simulink model "test_compare"  (R2023a)
settings: Solver=FixedStepAuto  StartTime=0.0  StopTime=10.0  FixedStep=0.002  RelTol=1e-3
PreLoadFcn:
  | xt = importrobot('urdf\XT_PRU_noHands.urdf', 'MaxNumBodies', 25);
  | xt.DataFormat = 'col';
  | 
  | urdfPath = "urdf/XT_PRU_noHands.urdf";
libraries: RoboticsCode x100, robotmaniplib x50
(part 1 of 2)
settings Model: Creator=kgross  LastModifiedBy=speedgoat
settings SolverCC: ConcurrentTasks=on  PositivePriorityOrder=on  AutoInsertRateTranBlk=on
settings OptimizationCC: BlockReduction=off  OptimizeBlockIOStorage=off
settings DebuggingCC: TasksWithSamePriorityMsg=none
settings HardwareCC: ProdBitPerLong=64  ProdLongLongMode=on  ProdHWDeviceType=Intel->x86-64 (Linux 64)
settings SFSimCC: SimTargetLang=C++
settings RTWCC: Description=Simulink Real-Time  SystemTargetFile=slrealtime.tlc  TemplateMakefile=slrealtime_default_tmf  Toolchain=Simulink Real-Time Toolchain  BuildConfiguration=Faster Runs  CodeExecutionProfiling=on  TargetLang=C++

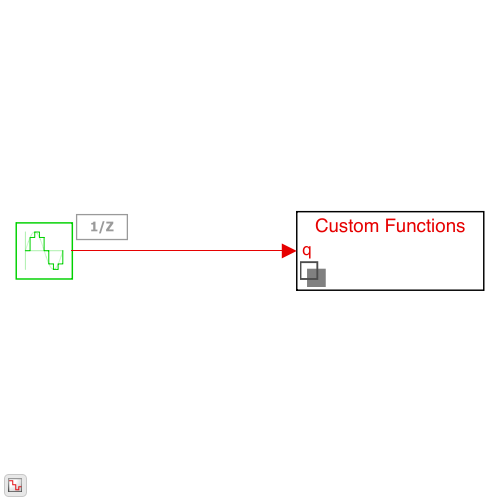
[thumbnail: Simulink's stored preview of the top-level diagram]
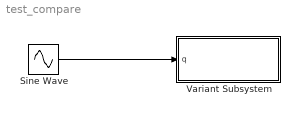
== system test_compare ==
  Sine Wave : Sin  Amplitude=1:16  Frequency=1:16  SampleTime=1
  Variant Subsystem : Subsystem  Variant=on  VariantControlMode=label  LabelModeActiveChoice=Custom
  wires:
  Sine Wave/1 -> Variant Subsystem/1(q)

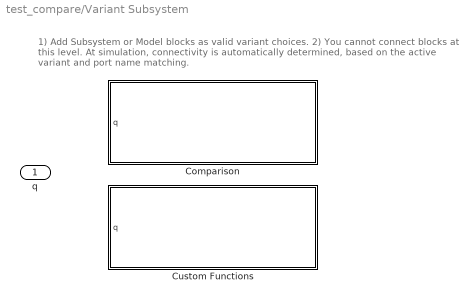
== system test_compare/Variant Subsystem ==
  note: 1) Add Subsystem or Model blocks as valid variant choices.
      | 2) You cannot connect blocks at this level. At simulation, connectivity is automatically
      | determined, based on the active variant and port name matching.
  q : Inport
  Comparison : Subsystem  VariantControl=Comparison
  Custom Functions : Subsystem  VariantControl=Custom

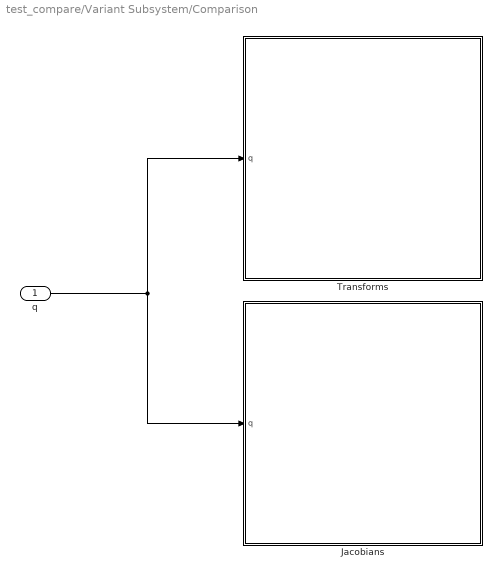
== system test_compare/Variant Subsystem/Comparison ==
  q : Inport
  Jacobians : Subsystem  VariantControl=Choice
  Transforms : Subsystem  VariantControl=Choice_1
  wires:
  q/1 -> Transforms/1(q), Jacobians/1(q)

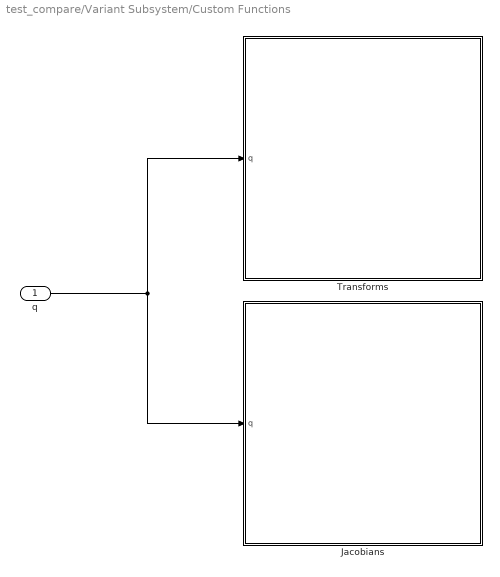
== system test_compare/Variant Subsystem/Custom Functions ==
  q : Inport
  Jacobians : Subsystem  VariantControl=Choice
  Transforms : Subsystem  VariantControl=Choice_1
  wires:
  q/1 -> Jacobians/1(q), Transforms/1(q)

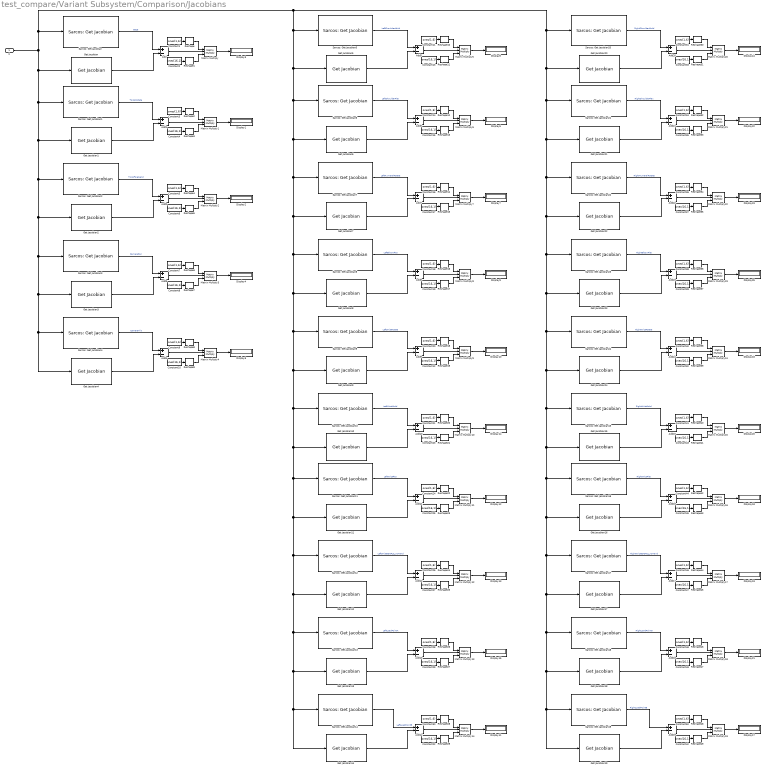
== system test_compare/Variant Subsystem/Comparison/Jacobians ==
  q : Inport
  Add{,1..24} (25 alike) : Sum  Inputs=+-
  Constant{1,3,5,7,9,11,14,16,18,20..21,24,26,28,30..31,34,36,38,40..41,44,46,48,50} (25 alike) : Constant  Value=ones(1,6)
  Constant{2,4,6,8,10,12..13,15,17,19,22..23,25,27,29,32..33,35,37,39,42..43,45,47,49} (25 alike) : Constant  Value=ones(16,1)
  Display{1..25} (25 alike) : Display
  Get Jacobian : robotmaniplib/Get Jacobian  RigidBodyTree=xt  EndEffector=Base  SimulateUsing=Interpreted execution
  Get Jacobian1 : robotmaniplib/Get Jacobian  RigidBodyTree=xt  EndEffector=TorsoRotate  SimulateUsing=Interpreted execution
  Get Jacobian10 : robotmaniplib/Get Jacobian  RigidBodyTree=xt  EndEffector=LeftWristAbAd  SimulateUsing=Interpreted execution
  Get Jacobian11 : robotmaniplib/Get Jacobian  RigidBodyTree=xt  EndEffector=LeftWristFlex  SimulateUsing=Interpreted execution
  Get Jacobian12 : robotmaniplib/Get Jacobian  RigidBodyTree=xt  EndEffector=LeftWrist6DOFLC_noHand  SimulateUsing=Interpreted execution
  Get Jacobian13 : robotmaniplib/Get Jacobian  RigidBodyTree=xt  EndEffector=LeftLoadPointA  SimulateUsing=Interpreted execution
  Get Jacobian14 : robotmaniplib/Get Jacobian  RigidBodyTree=xt  EndEffector=LeftLoadPointB  SimulateUsing=Interpreted execution
  Get Jacobian15 : robotmaniplib/Get Jacobian  RigidBodyTree=xt  EndEffector=RightWristAbAd  SimulateUsing=Interpreted execution
  Get Jacobian16 : robotmaniplib/Get Jacobian  RigidBodyTree=xt  EndEffector=RightWristFlex  SimulateUsing=Interpreted execution
  Get Jacobian17 : robotmaniplib/Get Jacobian  RigidBodyTree=xt  EndEffector=RightWrist6DOFLC_noHand  SimulateUsing=Interpreted execution
  Get Jacobian18 : robotmaniplib/Get Jacobian  RigidBodyTree=xt  EndEffector=RightLoadPointA  SimulateUsing=Interpreted execution
  Get Jacobian19 : robotmaniplib/Get Jacobian  RigidBodyTree=xt  EndEffector=RightLoadPointB  SimulateUsing=Interpreted execution
  Get Jacobian2 : robotmaniplib/Get Jacobian  RigidBodyTree=xt  EndEffector=TorsoForebend  SimulateUsing=Interpreted execution
  Get Jacobian20 : robotmaniplib/Get Jacobian  RigidBodyTree=xt  EndEffector=RightShoulderAbAd  SimulateUsing=Interpreted execution
  Get Jacobian21 : robotmaniplib/Get Jacobian  RigidBodyTree=xt  EndEffector=RightShoulderFlex  SimulateUsing=Interpreted execution
  Get Jacobian22 : robotmaniplib/Get Jacobian  RigidBodyTree=xt  EndEffector=RightHumeralRotate  SimulateUsing=Interpreted execution
  Get Jacobian23 : robotmaniplib/Get Jacobian  RigidBodyTree=xt  EndEffector=RightElbowFlex  SimulateUsing=Interpreted execution
  Get Jacobian24 : robotmaniplib/Get Jacobian  RigidBodyTree=xt  EndEffector=RightWristRotate  SimulateUsing=Interpreted execution
  Get Jacobian3 : robotmaniplib/Get Jacobian  RigidBodyTree=xt  EndEffector=CameraPan  SimulateUsing=Interpreted execution
  Get Jacobian4 : robotmaniplib/Get Jacobian  RigidBodyTree=xt  EndEffector=CameraTilt  SimulateUsing=Interpreted execution
  Get Jacobian5 : robotmaniplib/Get Jacobian  RigidBodyTree=xt  EndEffector=LeftShoulderAbAd  SimulateUsing=Interpreted execution
  Get Jacobian6 : robotmaniplib/Get Jacobian  RigidBodyTree=xt  EndEffector=LeftShoulderFlex  SimulateUsing=Interpreted execution
  Get Jacobian7 : robotmaniplib/Get Jacobian  RigidBodyTree=xt  EndEffector=LeftHumeralRotate  SimulateUsing=Interpreted execution
  Get Jacobian8 : robotmaniplib/Get Jacobian  RigidBodyTree=xt  EndEffector=LeftElbowFlex  SimulateUsing=Interpreted execution
  Get Jacobian9 : robotmaniplib/Get Jacobian  RigidBodyTree=xt  EndEffector=LeftWristRotate  SimulateUsing=Interpreted execution
  Matrix Multiply{,1..24} (25 alike) : Product  Inputs=3  Multiplication=Matrix(*)
  Reshape{,2,4,6,8,10,12,14,16,18,20,22,24,26,28,30,32,34,36,38,40,42,44,46,48} (25 alike) : Reshape  OutputDimensionality=Row vector (2-D)
  Reshape{1,3,5,7,9,11,13,15,17,19,21,23,25,27,29,31,33,35,37,39,41,43,45,47,49} (25 alike) : Reshape  OutputDimensionality=Column vector (2-D)
  Sarcos: Get Jacobian : RoboticsCode/Sarcos: Get Jacobian  urdfpath='XT_PRU_noHands.urdf'  source=Base  source_string='Base'  names_length=16
      settings: SourceProductName=Sacros Robotics Toolbox
  Sarcos: Get Jacobian1 : RoboticsCode/Sarcos: Get Jacobian  urdfpath='XT_PRU_noHands.urdf'  source=TorsoRotate  source_string='TorsoRotate'  names_length=16
      settings: SourceProductName=Sacros Robotics Toolbox
  Sarcos: Get Jacobian10 : RoboticsCode/Sarcos: Get Jacobian  urdfpath='XT_PRU_noHands.urdf'  source=LeftWristAbAd  source_string='LeftWristAbAd'  names_length=16
      settings: SourceProductName=Sacros Robotics Toolbox
  Sarcos: Get Jacobian11 : RoboticsCode/Sarcos: Get Jacobian  urdfpath='XT_PRU_noHands.urdf'  source=LeftWristFlex  source_string='LeftWristFlex'  names_length=16
      settings: SourceProductName=Sacros Robotics Toolbox
  Sarcos: Get Jacobian12 : RoboticsCode/Sarcos: Get Jacobian  urdfpath='XT_PRU_noHands.urdf'  source=LeftWrist6DOFLC_noHand  source_string='LeftWrist6DOFLC_noHand'  names_length=16
      settings: SourceProductName=Sacros Robotics Toolbox
  Sarcos: Get Jacobian13 : RoboticsCode/Sarcos: Get Jacobian  urdfpath='XT_PRU_noHands.urdf'  source=LeftLoadPointA  source_string='LeftLoadPointA'  names_length=16
      settings: SourceProductName=Sacros Robotics Toolbox
  Sarcos: Get Jacobian14 : RoboticsCode/Sarcos: Get Jacobian  urdfpath='XT_PRU_noHands.urdf'  source=LeftLoadPointB  source_string='LeftLoadPointB'  names_length=16
      settings: SourceProductName=Sacros Robotics Toolbox
  Sarcos: Get Jacobian15 : RoboticsCode/Sarcos: Get Jacobian  urdfpath='XT_PRU_noHands.urdf'  source=RightWristAbAd  source_string='RightWristAbAd'  names_length=16
      settings: SourceProductName=Sacros Robotics Toolbox
  Sarcos: Get Jacobian16 : RoboticsCode/Sarcos: Get Jacobian  urdfpath='XT_PRU_noHands.urdf'  source=RightWristFlex  source_string='RightWristFlex'  names_length=16
      settings: SourceProductName=Sacros Robotics Toolbox
  Sarcos: Get Jacobian17 : RoboticsCode/Sarcos: Get Jacobian  urdfpath='XT_PRU_noHands.urdf'  source=RightWrist6DOFLC_noHand  source_string='RightWrist6DOFLC_noHand'  names_length=16
      settings: SourceProductName=Sacros Robotics Toolbox
  Sarcos: Get Jacobian18 : RoboticsCode/Sarcos: Get Jacobian  urdfpath='XT_PRU_noHands.urdf'  source=RightLoadPointA  source_string='RightLoadPointA'  names_length=16
      settings: SourceProductName=Sacros Robotics Toolbox
  Sarcos: Get Jacobian19 : RoboticsCode/Sarcos: Get Jacobian  urdfpath='XT_PRU_noHands.urdf'  source=RightLoadPointB  source_string='RightLoadPointB'  names_length=16
      settings: SourceProductName=Sacros Robotics Toolbox
  Sarcos: Get Jacobian2 : RoboticsCode/Sarcos: Get Jacobian  urdfpath='XT_PRU_noHands.urdf'  source=TorsoForebend  source_string='TorsoForebend'  names_length=16
      settings: SourceProductName=Sacros Robotics Toolbox
  Sarcos: Get Jacobian20 : RoboticsCode/Sarcos: Get Jacobian  urdfpath='XT_PRU_noHands.urdf'  source=RightShoulderAbAd  source_string='RightShoulderAbAd'  names_length=16
      settings: SourceProductName=Sacros Robotics Toolbox
  Sarcos: Get Jacobian21 : RoboticsCode/Sarcos: Get Jacobian  urdfpath='XT_PRU_noHands.urdf'  source=RightShoulderFlex  source_string='RightShoulderFlex'  names_length=16
      settings: SourceProductName=Sacros Robotics Toolbox
  Sarcos: Get Jacobian22 : RoboticsCode/Sarcos: Get Jacobian  urdfpath='XT_PRU_noHands.urdf'  source=RightHumeralRotate  source_string='RightHumeralRotate'  names_length=16
      settings: SourceProductName=Sacros Robotics Toolbox
  Sarcos: Get Jacobian23 : RoboticsCode/Sarcos: Get Jacobian  urdfpath='XT_PRU_noHands.urdf'  source=RightElbowFlex  source_string='RightElbowFlex'  names_length=16
      settings: SourceProductName=Sacros Robotics Toolbox
  Sarcos: Get Jacobian24 : RoboticsCode/Sarcos: Get Jacobian  urdfpath='XT_PRU_noHands.urdf'  source=RightWristRotate  source_string='RightWristRotate'  names_length=16
      settings: SourceProductName=Sacros Robotics Toolbox
  Sarcos: Get Jacobian3 : RoboticsCode/Sarcos: Get Jacobian  urdfpath='XT_PRU_noHands.urdf'  source=CameraPan  source_string='CameraPan'  names_length=16
      settings: SourceProductName=Sacros Robotics Toolbox
  Sarcos: Get Jacobian4 : RoboticsCode/Sarcos: Get Jacobian  urdfpath='XT_PRU_noHands.urdf'  source=CameraTilt  source_string='CameraTilt'  names_length=16
      settings: SourceProductName=Sacros Robotics Toolbox
  Sarcos: Get Jacobian5 : RoboticsCode/Sarcos: Get Jacobian  urdfpath='XT_PRU_noHands.urdf'  source=LeftShoulderAbAd  source_string='LeftShoulderAbAd'  names_length=16
      settings: SourceProductName=Sacros Robotics Toolbox
  Sarcos: Get Jacobian6 : RoboticsCode/Sarcos: Get Jacobian  urdfpath='XT_PRU_noHands.urdf'  source=LeftShoulderFlex  source_string='LeftShoulderFlex'  names_length=16
      settings: SourceProductName=Sacros Robotics Toolbox
  Sarcos: Get Jacobian7 : RoboticsCode/Sarcos: Get Jacobian  urdfpath='XT_PRU_noHands.urdf'  source=LeftHumeralRotate  source_string='LeftHumeralRotate'  names_length=16
      settings: SourceProductName=Sacros Robotics Toolbox
  Sarcos: Get Jacobian8 : RoboticsCode/Sarcos: Get Jacobian  urdfpath='XT_PRU_noHands.urdf'  source=LeftElbowFlex  source_string='LeftElbowFlex'  names_length=16
      settings: SourceProductName=Sacros Robotics Toolbox
  Sarcos: Get Jacobian9 : RoboticsCode/Sarcos: Get Jacobian  urdfpath='XT_PRU_noHands.urdf'  source=LeftWristRotate  source_string='LeftWristRotate'  names_length=16
      settings: SourceProductName=Sacros Robotics Toolbox
  wires:
  Reshape1/1 -> Matrix Multiply/3
  Reshape/1 -> Matrix Multiply/1
  Constant2/1 -> Reshape1/1
  Matrix Multiply/1 -> Display3/1
  Constant1/1 -> Reshape/1
  Get Jacobian/1 -> Add/2
  Sarcos: Get Jacobian/1 -> Add/1  "Base"
  Add/1 -> Matrix Multiply/2
  Add1/1 -> Matrix Multiply1/2
  Sarcos: Get Jacobian1/1 -> Add1/1  "TorsoRotate"
  Get Jacobian1/1 -> Add1/2
  Constant3/1 -> Reshape2/1
  Matrix Multiply1/1 -> Display1/1
  Constant4/1 -> Reshape3/1
  Reshape2/1 -> Matrix Multiply1/1
  Reshape3/1 -> Matrix Multiply1/3
  Reshape5/1 -> Matrix Multiply2/3
  Reshape4/1 -> Matrix Multiply2/1
  Constant6/1 -> Reshape5/1
  Matrix Multiply2/1 -> Display2/1
  Constant5/1 -> Reshape4/1
  Get Jacobian2/1 -> Add2/2
  Sarcos: Get Jacobian2/1 -> Add2/1  "TorsoForebend"
  Add2/1 -> Matrix Multiply2/2
  Add3/1 -> Matrix Multiply3/2
  Sarcos: Get Jacobian3/1 -> Add3/1  "CameraPan"
  Get Jacobian3/1 -> Add3/2
  Constant7/1 -> Reshape6/1
  Matrix Multiply3/1 -> Display4/1
  Constant8/1 -> Reshape7/1
  Reshape6/1 -> Matrix Multiply3/1
  Reshape7/1 -> Matrix Multiply3/3
  Reshape9/1 -> Matrix Multiply4/3
  Reshape8/1 -> Matrix Multiply4/1
  Constant10/1 -> Reshape9/1
  Matrix Multiply4/1 -> Display5/1
  Constant9/1 -> Reshape8/1
  Get Jacobian4/1 -> Add4/2
  Sarcos: Get Jacobian4/1 -> Add4/1  "CameraTilt"
  Add4/1 -> Matrix Multiply4/2
  Add9/1 -> Matrix Multiply9/2
  Sarcos: Get Jacobian9/1 -> Add9/1  "LeftWristRotate"
  Get Jacobian9/1 -> Add9/2
  Constant20/1 -> Reshape18/1
  Matrix Multiply9/1 -> Display10/1
  Constant12/1 -> Reshape19/1
  Reshape18/1 -> Matrix Multiply9/1
  Reshape19/1 -> Matrix Multiply9/3
  Reshape17/1 -> Matrix Multiply8/3
  Reshape16/1 -> Matrix Multiply8/1
  Constant19/1 -> Reshape17/1
  Matrix Multiply8/1 -> Display9/1
  Constant18/1 -> Reshape16/1
  Get Jacobian8/1 -> Add8/2
  Sarcos: Get Jacobian8/1 -> Add8/1  "LeftElbowFlex"
  Add8/1 -> Matrix Multiply8/2
  Add7/1 -> Matrix Multiply7/2
  Sarcos: Get Jacobian7/1 -> Add7/1  "LeftHumeralRotate"
  Get Jacobian7/1 -> Add7/2
  Constant16/1 -> Reshape14/1
  Matrix Multiply7/1 -> Display7/1
  Constant17/1 -> Reshape15/1
  Reshape14/1 -> Matrix Multiply7/1
  Reshape15/1 -> Matrix Multiply7/3
  Reshape13/1 -> Matrix Multiply6/3
  Reshape12/1 -> Matrix Multiply6/1
  Constant15/1 -> Reshape13/1
  Matrix Multiply6/1 -> Display6/1
  Constant14/1 -> Reshape12/1
  Get Jacobian6/1 -> Add6/2
  Sarcos: Get Jacobian6/1 -> Add6/1  "LeftShoulderFlex"
  Add6/1 -> Matrix Multiply6/2
  Add5/1 -> Matrix Multiply5/2
  Sarcos: Get Jacobian5/1 -> Add5/1  "LeftShoulderAbAd"
  Get Jacobian5/1 -> Add5/2
  Constant11/1 -> Reshape10/1
  Matrix Multiply5/1 -> Display8/1
  Constant13/1 -> Reshape11/1
  Reshape10/1 -> Matrix Multiply5/1
  Reshape11/1 -> Matrix Multiply5/3
  Constant30/1 -> Reshape28/1
  Reshape27/1 -> Matrix Multiply13/3
  Get Jacobian14/1 -> Add14/2
  Reshape21/1 -> Matrix Multiply10/3
  Constant21/1 -> Reshape20/1
  Get Jacobian10/1 -> Add10/2
  Constant23/1 -> Reshape21/1
  Sarcos: Get Jacobian10/1 -> Add10/1  "LeftWristAbAd"
  Matrix Multiply10/1 -> Display14/1
  Add11/1 -> Matrix Multiply11/2
  Reshape29/1 -> Matrix Multiply14/3
  Constant24/1 -> Reshape22/1
  Reshape20/1 -> Matrix Multiply10/1
  Sarcos: Get Jacobian11/1 -> Add11/1  "LeftWristFlex"
  Get Jacobian11/1 -> Add11/2
  Constant25/1 -> Reshape23/1
  Reshape24/1 -> Matrix Multiply12/1
  Reshape22/1 -> Matrix Multiply11/1
  Reshape25/1 -> Matrix Multiply12/3
  Reshape23/1 -> Matrix Multiply11/3
  Constant27/1 -> Reshape25/1
  Reshape28/1 -> Matrix Multiply14/1
  Matrix Multiply12/1 -> Display13/1
  Reshape26/1 -> Matrix Multiply13/1
  Add12/1 -> Matrix Multiply12/2
  Get Jacobian12/1 -> Add12/2
  Matrix Multiply11/1 -> Display12/1
  Sarcos: Get Jacobian14/1 -> Add14/1  "LeftLoadPointB"
  Constant22/1 -> Reshape29/1
  Sarcos: Get Jacobian12/1 -> Add12/1  "LeftWrist6DOFLC_noHand"
  Matrix Multiply13/1 -> Display15/1
  Constant28/1 -> Reshape26/1
  Sarcos: Get Jacobian13/1 -> Add13/1  "LeftLoadPointA"
  Matrix Multiply14/1 -> Display11/1
  Get Jacobian13/1 -> Add13/2
  Add14/1 -> Matrix Multiply14/2
  Constant29/1 -> Reshape27/1
  Constant26/1 -> Reshape24/1
  Add13/1 -> Matrix Multiply13/2
  Add10/1 -> Matrix Multiply10/2
  Add15/1 -> Matrix Multiply15/2
  Add18/1 -> Matrix Multiply18/2
  Constant46/1 -> Reshape44/1
  Constant49/1 -> Reshape47/1
  Add19/1 -> Matrix Multiply19/2
  Get Jacobian18/1 -> Add18/2
  Matrix Multiply19/1 -> Display17/1
  Sarcos: Get Jacobian18/1 -> Add18/1  "RightLoadPointA"
  Constant48/1 -> Reshape46/1
  Matrix Multiply18/1 -> Display21/1
  Sarcos: Get Jacobian17/1 -> Add17/1  "RightWrist6DOFLC_noHand"
  Constant42/1 -> Reshape49/1
  Sarcos: Get Jacobian19/1 -> Add19/1  "RightLoadPointB"
  Matrix Multiply16/1 -> Display18/1
  Get Jacobian17/1 -> Add17/2
  Add17/1 -> Matrix Multiply17/2
  Reshape46/1 -> Matrix Multiply18/1
  Matrix Multiply17/1 -> Display19/1
  Reshape48/1 -> Matrix Multiply19/1
  Constant47/1 -> Reshape45/1
  Reshape43/1 -> Matrix Multiply16/3
  Reshape45/1 -> Matrix Multiply17/3
  Reshape42/1 -> Matrix Multiply16/1
  Reshape44/1 -> Matrix Multiply17/1
  Constant45/1 -> Reshape43/1
  Get Jacobian16/1 -> Add16/2
  Sarcos: Get Jacobian16/1 -> Add16/1  "RightWristFlex"
  Reshape40/1 -> Matrix Multiply15/1
  Constant44/1 -> Reshape42/1
  Reshape49/1 -> Matrix Multiply19/3
  Add16/1 -> Matrix Multiply16/2
  Matrix Multiply15/1 -> Display20/1
  Sarcos: Get Jacobian15/1 -> Add15/1  "RightWristAbAd"
  Constant43/1 -> Reshape41/1
  Get Jacobian15/1 -> Add15/2
  Constant41/1 -> Reshape40/1
  Reshape41/1 -> Matrix Multiply15/3
  Get Jacobian19/1 -> Add19/2
  Reshape47/1 -> Matrix Multiply18/3
  Constant50/1 -> Reshape48/1
  q/1 -> Sarcos: Get Jacobian20/1, Get Jacobian21/1, Get Jacobian16/1, Get Jacobian19/1, Sarcos: Get Jacobian19/1, Get Jacobian18/1, Sarcos: Get Jacobian18/1, Get Jacobian17/1, Sarcos: Get Jacobian17/1, Sarcos: Get Jacobian16/1, Get Jacobian15/1, Sarcos: Get Jacobian15/1, Get Jacobian24/1, Sarcos: Get Jacobian24/1, Get Jacobian23/1, Sarcos: Get Jacobian23/1, Get Jacobian22/1, Sarcos: Get Jacobian22/1, Sarcos: Get Jacobian21/1, Get Jacobian20/1, Get Jacobian5/1, Sarcos: Get Jacobian6/1, Sarcos: Get Jacobian7/1, Get Jacobian7/1, Sarcos: Get Jacobian8/1, Get Jacobian8/1, Sarcos: Get Jacobian9/1, Get Jacobian9/1, Sarcos: Get Jacobian10/1, Get Jacobian10/1, Sarcos: Get Jacobian11/1, Sarcos: Get Jacobian12/1, Get Jacobian12/1, Sarcos: Get Jacobian13/1, Get Jacobian13/1, Sarcos: Get Jacobian14/1, Get Jacobian14/1, Get Jacobian11/1, Get Jacobian6/1, Sarcos: Get Jacobian5/1, Sarcos: Get Jacobian/1, Get Jacobian1/1, Get Jacobian4/1, Sarcos: Get Jacobian4/1, Get Jacobian3/1, Sarcos: Get Jacobian3/1, Get Jacobian2/1, Sarcos: Get Jacobian2/1, Sarcos: Get Jacobian1/1, Get Jacobian/1
  Reshape31/1 -> Matrix Multiply20/3
  Reshape30/1 -> Matrix Multiply20/1
  Constant33/1 -> Reshape31/1
  Matrix Multiply20/1 -> Display24/1
  Constant31/1 -> Reshape30/1
  Get Jacobian20/1 -> Add20/2
  Sarcos: Get Jacobian20/1 -> Add20/1  "RightShoulderAbAd"
  Add20/1 -> Matrix Multiply20/2
  Add21/1 -> Matrix Multiply21/2
  Sarcos: Get Jacobian21/1 -> Add21/1  "RightShoulderFlex"
  Get Jacobian21/1 -> Add21/2
  Constant34/1 -> Reshape32/1
  Matrix Multiply21/1 -> Display22/1
  Constant35/1 -> Reshape33/1
  Reshape32/1 -> Matrix Multiply21/1
  Reshape33/1 -> Matrix Multiply21/3
  Reshape35/1 -> Matrix Multiply22/3
  Reshape34/1 -> Matrix Multiply22/1
  Constant37/1 -> Reshape35/1
  Matrix Multiply22/1 -> Display23/1
  Constant36/1 -> Reshape34/1
  Get Jacobian22/1 -> Add22/2
  Sarcos: Get Jacobian22/1 -> Add22/1  "RightHumeralRotate"
  Add22/1 -> Matrix Multiply22/2
  Add23/1 -> Matrix Multiply23/2
  Sarcos: Get Jacobian23/1 -> Add23/1  "RightElbowFlex"
  Get Jacobian23/1 -> Add23/2
  Constant38/1 -> Reshape36/1
  Matrix Multiply23/1 -> Display25/1
  Constant39/1 -> Reshape37/1
  Reshape36/1 -> Matrix Multiply23/1
  Reshape37/1 -> Matrix Multiply23/3
  Reshape39/1 -> Matrix Multiply24/3
  Reshape38/1 -> Matrix Multiply24/1
  Constant32/1 -> Reshape39/1
  Matrix Multiply24/1 -> Display16/1
  Constant40/1 -> Reshape38/1
  Get Jacobian24/1 -> Add24/2
  Sarcos: Get Jacobian24/1 -> Add24/1  "RightWristRotate"
  Add24/1 -> Matrix Multiply24/2

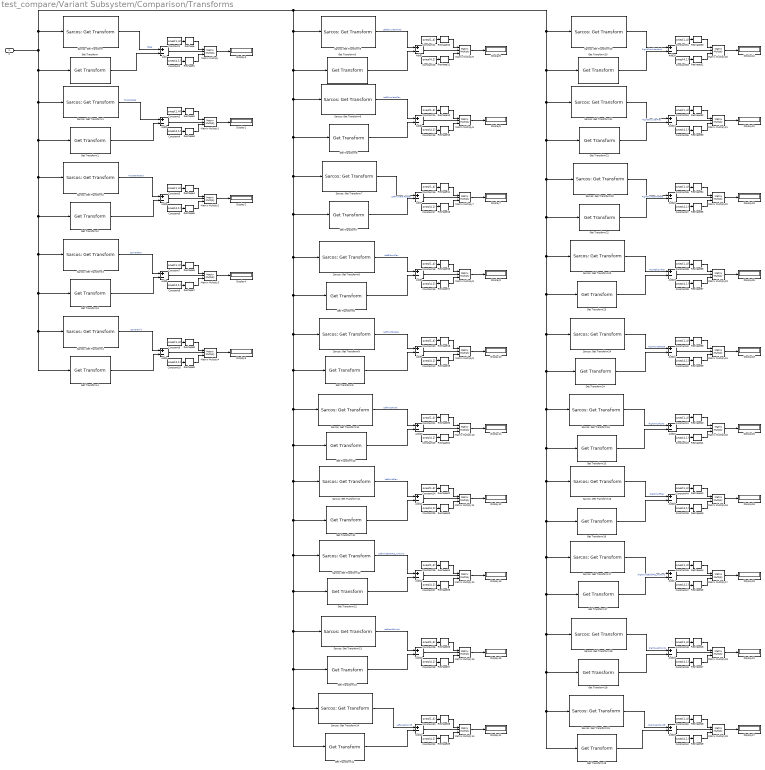
== system test_compare/Variant Subsystem/Comparison/Transforms ==
  q : Inport
  Add{,1..24} (25 alike) : Sum  Inputs=+-
  Constant{1,3,5,7,9,11,14,16,18,20..21,24,26,28,30..31,34,36,38,40..41,44,46,48,50} (25 alike) : Constant  Value=ones(1,4)
  Constant{2,4,6,8,10,12..13,15,17,19,22..23,25,27,29,32..33,35,37,39,42..43,45,47,49} (25 alike) : Constant  Value=ones(4,1)
  Display{1..25} (25 alike) : Display
  Get Transform : robotmaniplib/Get Transform  RigidBodyTree=xt  SourceBody=Base  TargetBody=World  SimulateUsing=Interpreted execution
  Get Transform1 : robotmaniplib/Get Transform  RigidBodyTree=xt  SourceBody=TorsoRotate  TargetBody=World  SimulateUsing=Interpreted execution
  Get Transform10 : robotmaniplib/Get Transform  RigidBodyTree=xt  SourceBody=LeftWristAbAd  TargetBody=World  SimulateUsing=Interpreted execution
  Get Transform11 : robotmaniplib/Get Transform  RigidBodyTree=xt  SourceBody=LeftWristFlex  TargetBody=World  SimulateUsing=Interpreted execution
  Get Transform12 : robotmaniplib/Get Transform  RigidBodyTree=xt  SourceBody=LeftWrist6DOFLC_noHand  TargetBody=World  SimulateUsing=Interpreted execution
  Get Transform13 : robotmaniplib/Get Transform  RigidBodyTree=xt  SourceBody=LeftLoadPointA  TargetBody=World  SimulateUsing=Interpreted execution
  Get Transform14 : robotmaniplib/Get Transform  RigidBodyTree=xt  SourceBody=LeftLoadPointB  TargetBody=World  SimulateUsing=Interpreted execution
  Get Transform15 : robotmaniplib/Get Transform  RigidBodyTree=xt  SourceBody=RightWristAbAd  TargetBody=World  SimulateUsing=Interpreted execution
  Get Transform16 : robotmaniplib/Get Transform  RigidBodyTree=xt  SourceBody=RightWristFlex  TargetBody=World  SimulateUsing=Interpreted execution
  Get Transform17 : robotmaniplib/Get Transform  RigidBodyTree=xt  SourceBody=RightWrist6DOFLC_noHand  TargetBody=World  SimulateUsing=Interpreted execution
  Get Transform18 : robotmaniplib/Get Transform  RigidBodyTree=xt  SourceBody=RightLoadPointA  TargetBody=World  SimulateUsing=Interpreted execution
  Get Transform19 : robotmaniplib/Get Transform  RigidBodyTree=xt  SourceBody=RightLoadPointB  TargetBody=World  SimulateUsing=Interpreted execution
  Get Transform2 : robotmaniplib/Get Transform  RigidBodyTree=xt  SourceBody=TorsoForebend  TargetBody=World  SimulateUsing=Interpreted execution
  Get Transform20 : robotmaniplib/Get Transform  RigidBodyTree=xt  SourceBody=RightShoulderAbAd  TargetBody=World  SimulateUsing=Interpreted execution
  Get Transform21 : robotmaniplib/Get Transform  RigidBodyTree=xt  SourceBody=RightShoulderFlex  TargetBody=World  SimulateUsing=Interpreted execution
  Get Transform22 : robotmaniplib/Get Transform  RigidBodyTree=xt  SourceBody=RightHumeralRotate  TargetBody=World  SimulateUsing=Interpreted execution
  Get Transform23 : robotmaniplib/Get Transform  RigidBodyTree=xt  SourceBody=RightElbowFlex  TargetBody=World  SimulateUsing=Interpreted execution
  Get Transform24 : robotmaniplib/Get Transform  RigidBodyTree=xt  SourceBody=RightWristRotate  TargetBody=World  SimulateUsing=Interpreted execution
  Get Transform3 : robotmaniplib/Get Transform  RigidBodyTree=xt  SourceBody=CameraPan  TargetBody=World  SimulateUsing=Interpreted execution
  Get Transform4 : robotmaniplib/Get Transform  RigidBodyTree=xt  SourceBody=CameraTilt  TargetBody=World  SimulateUsing=Interpreted execution
  Get Transform5 : robotmaniplib/Get Transform  RigidBodyTree=xt  SourceBody=LeftShoulderAbAd  TargetBody=World  SimulateUsing=Interpreted execution
  Get Transform6 : robotmaniplib/Get Transform  RigidBodyTree=xt  SourceBody=LeftShoulderFlex  TargetBody=World  SimulateUsing=Interpreted execution
  Get Transform7 : robotmaniplib/Get Transform  RigidBodyTree=xt  SourceBody=LeftHumeralRotate  TargetBody=World  SimulateUsing=Interpreted execution
  Get Transform8 : robotmaniplib/Get Transform  RigidBodyTree=xt  SourceBody=LeftElbowFlex  TargetBody=World  SimulateUsing=Interpreted execution
  Get Transform9 : robotmaniplib/Get Transform  RigidBodyTree=xt  SourceBody=LeftWristRotate  TargetBody=World  SimulateUsing=Interpreted execution
  Matrix Multiply{,1..24} (25 alike) : Product  Inputs=3  Multiplication=Matrix(*)
  Reshape{,2,4,6,8,10,12,14,16,18,20,22,24,26,28,30,32,34,36,38,40,42,44,46,48} (25 alike) : Reshape  OutputDimensionality=Row vector (2-D)
  Reshape{1,3,5,7,9,11,13,15,17,19,21,23,25,27,29,31,33,35,37,39,41,43,45,47,49} (25 alike) : Reshape  OutputDimensionality=Column vector (2-D)
  Sarcos: Get Transform : RoboticsCode/Sarcos: Get Transform  urdfpath='XT_PRU_noHands.urdf'  source=Base  source_string='Base'  target=World  target_string='World'
      settings: SourceProductName=Sacros Robotics Toolbox
  Sarcos: Get Transform1 : RoboticsCode/Sarcos: Get Transform  urdfpath='XT_PRU_noHands.urdf'  source=TorsoRotate  source_string='TorsoRotate'  target=World  target_string='World'
      settings: SourceProductName=Sacros Robotics Toolbox
  Sarcos: Get Transform10 : RoboticsCode/Sarcos: Get Transform  urdfpath='XT_PRU_noHands.urdf'  source=LeftWristAbAd  source_string='LeftWristAbAd'  target=World  target_string='World'
      settings: SourceProductName=Sacros Robotics Toolbox
  Sarcos: Get Transform11 : RoboticsCode/Sarcos: Get Transform  urdfpath='XT_PRU_noHands.urdf'  source=LeftWristFlex  source_string='LeftWristFlex'  target=World  target_string='World'
      settings: SourceProductName=Sacros Robotics Toolbox
  Sarcos: Get Transform12 : RoboticsCode/Sarcos: Get Transform  urdfpath='XT_PRU_noHands.urdf'  source=LeftWrist6DOFLC_noHand  source_string='LeftWrist6DOFLC_noHand'  target=World  target_string='World'
      settings: SourceProductName=Sacros Robotics Toolbox
  Sarcos: Get Transform13 : RoboticsCode/Sarcos: Get Transform  urdfpath='XT_PRU_noHands.urdf'  source=LeftLoadPointA  source_string='LeftLoadPointA'  target=World  target_string='World'
      settings: SourceProductName=Sacros Robotics Toolbox
  Sarcos: Get Transform14 : RoboticsCode/Sarcos: Get Transform  urdfpath='XT_PRU_noHands.urdf'  source=LeftLoadPointB  source_string='LeftLoadPointB'  target=World  target_string='World'
      settings: SourceProductName=Sacros Robotics Toolbox
  Sarcos: Get Transform15 : RoboticsCode/Sarcos: Get Transform  urdfpath='XT_PRU_noHands.urdf'  source=RightWristAbAd  source_string='RightWristAbAd'  target=World  target_string='World'
      settings: SourceProductName=Sacros Robotics Toolbox
  Sarcos: Get Transform16 : RoboticsCode/Sarcos: Get Transform  urdfpath='XT_PRU_noHands.urdf'  source=RightWristFlex  source_string='RightWristFlex'  target=World  target_string='World'
      settings: SourceProductName=Sacros Robotics Toolbox
  Sarcos: Get Transform17 : RoboticsCode/Sarcos: Get Transform  urdfpath='XT_PRU_noHands.urdf'  source=RightWrist6DOFLC_noHand  source_string='RightWrist6DOFLC_noHand'  target=World  target_string='World'
      settings: SourceProductName=Sacros Robotics Toolbox
  Sarcos: Get Transform18 : RoboticsCode/Sarcos: Get Transform  urdfpath='XT_PRU_noHands.urdf'  source=RightLoadPointA  source_string='RightLoadPointA'  target=World  target_string='World'
      settings: SourceProductName=Sacros Robotics Toolbox
  Sarcos: Get Transform19 : RoboticsCode/Sarcos: Get Transform  urdfpath='XT_PRU_noHands.urdf'  source=RightLoadPointB  source_string='RightLoadPointB'  target=World  target_string='World'
      settings: SourceProductName=Sacros Robotics Toolbox
  Sarcos: Get Transform2 : RoboticsCode/Sarcos: Get Transform  urdfpath='XT_PRU_noHands.urdf'  source=TorsoForebend  source_string='TorsoForebend'  target=World  target_string='World'
      settings: SourceProductName=Sacros Robotics Toolbox
  Sarcos: Get Transform20 : RoboticsCode/Sarcos: Get Transform  urdfpath='XT_PRU_noHands.urdf'  source=RightShoulderAbAd  source_string='RightShoulderAbAd'  target=World  target_string='World'
      settings: SourceProductName=Sacros Robotics Toolbox
  Sarcos: Get Transform21 : RoboticsCode/Sarcos: Get Transform  urdfpath='XT_PRU_noHands.urdf'  source=RightShoulderFlex  source_string='RightShoulderFlex'  target=World  target_string='World'
      settings: SourceProductName=Sacros Robotics Toolbox
  Sarcos: Get Transform22 : RoboticsCode/Sarcos: Get Transform  urdfpath='XT_PRU_noHands.urdf'  source=RightHumeralRotate  source_string='RightHumeralRotate'  target=World  target_string='World'
      settings: SourceProductName=Sacros Robotics Toolbox
  Sarcos: Get Transform23 : RoboticsCode/Sarcos: Get Transform  urdfpath='XT_PRU_noHands.urdf'  source=RightElbowFlex  source_string='RightElbowFlex'  target=World  target_string='World'
      settings: SourceProductName=Sacros Robotics Toolbox
  Sarcos: Get Transform24 : RoboticsCode/Sarcos: Get Transform  urdfpath='XT_PRU_noHands.urdf'  source=RightWristRotate  source_string='RightWristRotate'  target=World  target_string='World'
      settings: SourceProductName=Sacros Robotics Toolbox
  Sarcos: Get Transform3 : RoboticsCode/Sarcos: Get Transform  urdfpath='XT_PRU_noHands.urdf'  source=CameraPan  source_string='CameraPan'  target=World  target_string='World'
      settings: SourceProductName=Sacros Robotics Toolbox
  Sarcos: Get Transform4 : RoboticsCode/Sarcos: Get Transform  urdfpath='XT_PRU_noHands.urdf'  source=CameraTilt  source_string='CameraTilt'  target=World  target_string='World'
      settings: SourceProductName=Sacros Robotics Toolbox
  Sarcos: Get Transform5 : RoboticsCode/Sarcos: Get Transform  urdfpath='XT_PRU_noHands.urdf'  source=LeftShoulderAbAd  source_string='LeftShoulderAbAd'  target=World  target_string='World'
      settings: SourceProductName=Sacros Robotics Toolbox
  Sarcos: Get Transform6 : RoboticsCode/Sarcos: Get Transform  urdfpath='XT_PRU_noHands.urdf'  source=LeftShoulderFlex  source_string='LeftShoulderFlex'  target=World  target_string='World'
      settings: SourceProductName=Sacros Robotics Toolbox
  Sarcos: Get Transform7 : RoboticsCode/Sarcos: Get Transform  urdfpath='XT_PRU_noHands.urdf'  source=LeftHumeralRotate  source_string='LeftHumeralRotate'  target=World  target_string='World'
      settings: SourceProductName=Sacros Robotics Toolbox
  Sarcos: Get Transform8 : RoboticsCode/Sarcos: Get Transform  urdfpath='XT_PRU_noHands.urdf'  source=LeftElbowFlex  source_string='LeftElbowFlex'  target=World  target_string='World'
      settings: SourceProductName=Sacros Robotics Toolbox
  Sarcos: Get Transform9 : RoboticsCode/Sarcos: Get Transform  urdfpath='XT_PRU_noHands.urdf'  source=LeftWristRotate  source_string='LeftWristRotate'  target=World  target_string='World'
      settings: SourceProductName=Sacros Robotics Toolbox
  wires:
  Add24/1 -> Matrix Multiply24/2
  Sarcos: Get Transform24/1 -> Add24/1  "RightWristRotate"
  Get Transform24/1 -> Add24/2
  Constant40/1 -> Reshape38/1
  Matrix Multiply24/1 -> Display16/1
  Constant32/1 -> Reshape39/1
  Reshape38/1 -> Matrix Multiply24/1
  Reshape39/1 -> Matrix Multiply24/3
  Reshape37/1 -> Matrix Multiply23/3
  Reshape36/1 -> Matrix Multiply23/1
  Constant39/1 -> Reshape37/1
  Matrix Multiply23/1 -> Display25/1
  Constant38/1 -> Reshape36/1
  Get Transform23/1 -> Add23/2
  Sarcos: Get Transform23/1 -> Add23/1  "RightElbowFlex"
  Add23/1 -> Matrix Multiply23/2
  Add22/1 -> Matrix Multiply22/2
  Sarcos: Get Transform22/1 -> Add22/1  "RightHumeralRotate"
  Get Transform22/1 -> Add22/2
  Constant36/1 -> Reshape34/1
  Matrix Multiply22/1 -> Display23/1
  Constant37/1 -> Reshape35/1
  Reshape34/1 -> Matrix Multiply22/1
  Reshape35/1 -> Matrix Multiply22/3
  Reshape33/1 -> Matrix Multiply21/3
  Reshape32/1 -> Matrix Multiply21/1
  Constant35/1 -> Reshape33/1
  Matrix Multiply21/1 -> Display22/1
  Constant34/1 -> Reshape32/1
  Get Transform21/1 -> Add21/2
  Sarcos: Get Transform21/1 -> Add21/1  "RightShoulderFlex"
  Add21/1 -> Matrix Multiply21/2
  Add20/1 -> Matrix Multiply20/2
  Sarcos: Get Transform20/1 -> Add20/1  "RightShoulderAbAd"
  Get Transform20/1 -> Add20/2
  Constant31/1 -> Reshape30/1
  Matrix Multiply20/1 -> Display24/1
  Constant33/1 -> Reshape31/1
  Reshape30/1 -> Matrix Multiply20/1
  Reshape31/1 -> Matrix Multiply20/3
  q/1 -> Get Transform/1, Sarcos: Get Transform1/1, Get Transform1/1, Get Transform4/1, Sarcos: Get Transform4/1, Get Transform3/1, Sarcos: Get Transform3/1, Get Transform2/1, Sarcos: Get Transform2/1, Sarcos: Get Transform/1, Sarcos: Get Transform5/1, Get Transform5/1, Get Transform6/1, Sarcos: Get Transform7/1, Sarcos: Get Transform8/1, Get Transform8/1, Sarcos: Get Transform9/1, Get Transform9/1, Sarcos: Get Transform10/1, Sarcos: Get Transform11/1, Get Transform11/1, Sarcos: Get Transform12/1, Get Transform14/1, Sarcos: Get Transform14/1, Get Transform13/1, Sarcos: Get Transform13/1, Get Transform12/1, Get Transform10/1, Get Transform7/1, Sarcos: Get Transform6/1, Sarcos: Get Transform20/1, Get Transform20/1, Sarcos: Get Transform21/1, Get Transform21/1, Sarcos: Get Transform22/1, Get Transform22/1, Sarcos: Get Transform24/1, Sarcos: Get Transform15/1, Get Transform15/1, Sarcos: Get Transform16/1, Sarcos: Get Transform17/1, Sarcos: Get Transform18/1, Get Transform18/1, Get Transform19/1, Sarcos: Get Transform19/1, Get Transform17/1, Get Transform16/1, Get Transform24/1, Get Transform23/1, Sarcos: Get Transform23/1
  Constant50/1 -> Reshape48/1
  Reshape47/1 -> Matrix Multiply18/3
  Get Transform19/1 -> Add19/2
  Reshape41/1 -> Matrix Multiply15/3
  Constant41/1 -> Reshape40/1
  Get Transform15/1 -> Add15/2
  Constant43/1 -> Reshape41/1
  Sarcos: Get Transform15/1 -> Add15/1  "RightWristAbAd"
  Matrix Multiply15/1 -> Display20/1
  Add16/1 -> Matrix Multiply16/2
  Reshape49/1 -> Matrix Multiply19/3
  Constant44/1 -> Reshape42/1
  Reshape40/1 -> Matrix Multiply15/1
  Sarcos: Get Transform16/1 -> Add16/1  "RightWristFlex"
  Get Transform16/1 -> Add16/2
  Constant45/1 -> Reshape43/1
  Reshape44/1 -> Matrix Multiply17/1
  Reshape42/1 -> Matrix Multiply16/1
  Reshape45/1 -> Matrix Multiply17/3
  Reshape43/1 -> Matrix Multiply16/3
  Constant47/1 -> Reshape45/1
  Reshape48/1 -> Matrix Multiply19/1
  Matrix Multiply17/1 -> Display19/1
  Reshape46/1 -> Matrix Multiply18/1
  Add17/1 -> Matrix Multiply17/2
  Get Transform17/1 -> Add17/2
  Matrix Multiply16/1 -> Display18/1
  Sarcos: Get Transform19/1 -> Add19/1  "RightLoadPointB"
  Constant42/1 -> Reshape49/1
  Sarcos: Get Transform17/1 -> Add17/1  "RightWrist6DOFLC_noHand"
  Matrix Multiply18/1 -> Display21/1
  Constant48/1 -> Reshape46/1
  Sarcos: Get Transform18/1 -> Add18/1  "RightLoadPointA"
  Matrix Multiply19/1 -> Display17/1
  Get Transform18/1 -> Add18/2
  Add19/1 -> Matrix Multiply19/2
  Constant49/1 -> Reshape47/1
  Constant46/1 -> Reshape44/1
  Add18/1 -> Matrix Multiply18/2
  Add15/1 -> Matrix Multiply15/2
  Add10/1 -> Matrix Multiply10/2
  Add13/1 -> Matrix Multiply13/2
  Constant26/1 -> Reshape24/1
  Constant29/1 -> Reshape27/1
  Add14/1 -> Matrix Multiply14/2
  Get Transform13/1 -> Add13/2
  Matrix Multiply14/1 -> Display11/1
  Sarcos: Get Transform13/1 -> Add13/1  "LeftLoadPointA"
  Constant28/1 -> Reshape26/1
  Matrix Multiply13/1 -> Display15/1
  Sarcos: Get Transform12/1 -> Add12/1  "LeftWrist6DOFLC_noHand"
  Constant22/1 -> Reshape29/1
  Sarcos: Get Transform14/1 -> Add14/1  "LeftLoadPointB"
  Matrix Multiply11/1 -> Display12/1
  Get Transform12/1 -> Add12/2
  Add12/1 -> Matrix Multiply12/2
  Reshape26/1 -> Matrix Multiply13/1
  Matrix Multiply12/1 -> Display13/1
  Reshape28/1 -> Matrix Multiply14/1
  Constant27/1 -> Reshape25/1
  Reshape23/1 -> Matrix Multiply11/3
  Reshape25/1 -> Matrix Multiply12/3
  Reshape22/1 -> Matrix Multiply11/1
  Reshape24/1 -> Matrix Multiply12/1
  Constant25/1 -> Reshape23/1
  Get Transform11/1 -> Add11/2
  Sarcos: Get Transform11/1 -> Add11/1  "LeftWristFlex"
  Reshape20/1 -> Matrix Multiply10/1
  Constant24/1 -> Reshape22/1
  Reshape29/1 -> Matrix Multiply14/3
  Add11/1 -> Matrix Multiply11/2
  Matrix Multiply10/1 -> Display14/1
  Sarcos: Get Transform10/1 -> Add10/1  "LeftWristAbAd"
  Constant23/1 -> Reshape21/1
  Get Transform10/1 -> Add10/2
  Constant21/1 -> Reshape20/1
  Reshape21/1 -> Matrix Multiply10/3
  Get Transform14/1 -> Add14/2
  Reshape27/1 -> Matrix Multiply13/3
  Constant30/1 -> Reshape28/1
  Reshape11/1 -> Matrix Multiply5/3
  Reshape10/1 -> Matrix Multiply5/1
  Constant13/1 -> Reshape11/1
  Matrix Multiply5/1 -> Display8/1
  Constant11/1 -> Reshape10/1
  Get Transform5/1 -> Add5/2
  Sarcos: Get Transform5/1 -> Add5/1  "LeftShoulderAbAd"
  Add5/1 -> Matrix Multiply5/2
  Add6/1 -> Matrix Multiply6/2
  Sarcos: Get Transform6/1 -> Add6/1  "LeftShoulderFlex"
  Get Transform6/1 -> Add6/2
  Constant14/1 -> Reshape12/1
  Matrix Multiply6/1 -> Display6/1
  Constant15/1 -> Reshape13/1
  Reshape12/1 -> Matrix Multiply6/1
  Reshape13/1 -> Matrix Multiply6/3
  Reshape15/1 -> Matrix Multiply7/3
  Reshape14/1 -> Matrix Multiply7/1
  Constant17/1 -> Reshape15/1
  Matrix Multiply7/1 -> Display7/1
  Constant16/1 -> Reshape14/1
  Get Transform7/1 -> Add7/2
  Sarcos: Get Transform7/1 -> Add7/1  "LeftHumeralRotate"
  Add7/1 -> Matrix Multiply7/2
  Add8/1 -> Matrix Multiply8/2
  Sarcos: Get Transform8/1 -> Add8/1  "LeftElbowFlex"
  Get Transform8/1 -> Add8/2
  Constant18/1 -> Reshape16/1
  Matrix Multiply8/1 -> Display9/1
  Constant19/1 -> Reshape17/1
  Reshape16/1 -> Matrix Multiply8/1
  Reshape17/1 -> Matrix Multiply8/3
  Reshape19/1 -> Matrix Multiply9/3
  Reshape18/1 -> Matrix Multiply9/1
  Constant12/1 -> Reshape19/1
  Matrix Multiply9/1 -> Display10/1
  Constant20/1 -> Reshape18/1
  Get Transform9/1 -> Add9/2
  Sarcos: Get Transform9/1 -> Add9/1  "LeftWristRotate"
  Add9/1 -> Matrix Multiply9/2
  Add4/1 -> Matrix Multiply4/2
  Sarcos: Get Transform4/1 -> Add4/1  "CameraTilt"
  Get Transform4/1 -> Add4/2
  Constant9/1 -> Reshape8/1
  Matrix Multiply4/1 -> Display5/1
  Constant10/1 -> Reshape9/1
  Reshape8/1 -> Matrix Multiply4/1
  Reshape9/1 -> Matrix Multiply4/3
  Reshape7/1 -> Matrix Multiply3/3
  Reshape6/1 -> Matrix Multiply3/1
  Constant8/1 -> Reshape7/1
  Matrix Multiply3/1 -> Display4/1
  Constant7/1 -> Reshape6/1
  Get Transform3/1 -> Add3/2
  Sarcos: Get Transform3/1 -> Add3/1  "CameraPan"
  Add3/1 -> Matrix Multiply3/2
  Add2/1 -> Matrix Multiply2/2
  Sarcos: Get Transform2/1 -> Add2/1  "TorsoForebend"
  Get Transform2/1 -> Add2/2
  Constant5/1 -> Reshape4/1
  Matrix Multiply2/1 -> Display2/1
  Constant6/1 -> Reshape5/1
  Reshape4/1 -> Matrix Multiply2/1
  Reshape5/1 -> Matrix Multiply2/3
  Reshape3/1 -> Matrix Multiply1/3
  Reshape2/1 -> Matrix Multiply1/1
  Constant4/1 -> Reshape3/1
  Matrix Multiply1/1 -> Display1/1
  Constant3/1 -> Reshape2/1
  Get Transform1/1 -> Add1/2
  Sarcos: Get Transform1/1 -> Add1/1  "TorsoRotate"
  Add1/1 -> Matrix Multiply1/2
  Add/1 -> Matrix Multiply/2
  Sarcos: Get Transform/1 -> Add/1  "Base"
  Get Transform/1 -> Add/2
  Constant1/1 -> Reshape/1
  Matrix Multiply/1 -> Display3/1
  Constant2/1 -> Reshape1/1
  Reshape/1 -> Matrix Multiply/1
  Reshape1/1 -> Matrix Multiply/3

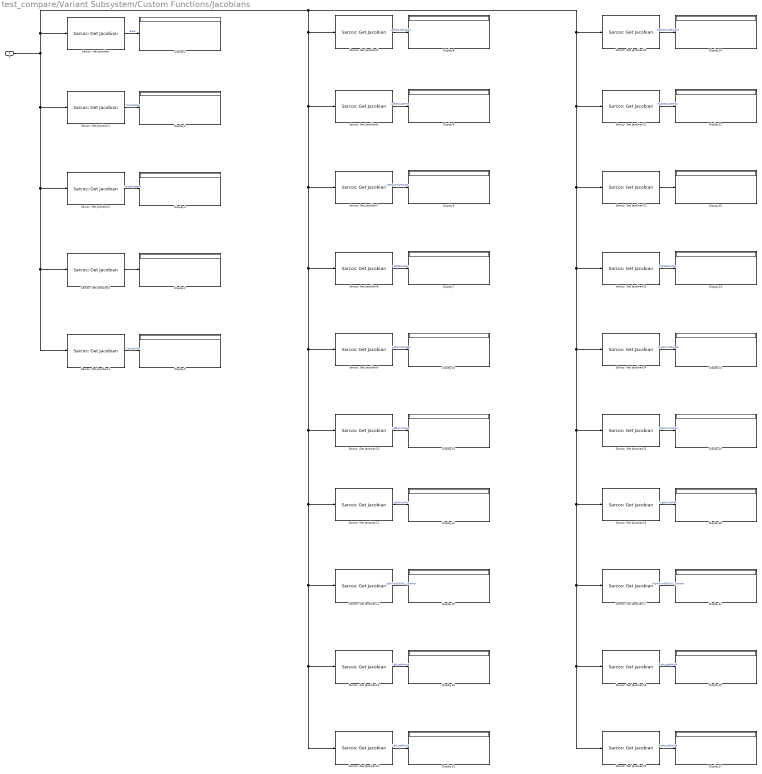
== system test_compare/Variant Subsystem/Custom Functions/Jacobians ==
  q : Inport
  Display{1..25} (25 alike) : Display
  Sarcos: Get Jacobian : RoboticsCode/Sarcos: Get Jacobian  urdfpath='XT_PRU_noHands.urdf'  source=Base  source_string='Base'  names_length=16
      settings: SourceProductName=Sacros Robotics Toolbox
  Sarcos: Get Jacobian1 : RoboticsCode/Sarcos: Get Jacobian  urdfpath='XT_PRU_noHands.urdf'  source=TorsoRotate  source_string='TorsoRotate'  names_length=16
      settings: SourceProductName=Sacros Robotics Toolbox
  Sarcos: Get Jacobian10 : RoboticsCode/Sarcos: Get Jacobian  urdfpath='XT_PRU_noHands.urdf'  source=LeftWristAbAd  source_string='LeftWristAbAd'  names_length=16
      settings: SourceProductName=Sacros Robotics Toolbox
  Sarcos: Get Jacobian11 : RoboticsCode/Sarcos: Get Jacobian  urdfpath='XT_PRU_noHands.urdf'  source=LeftWristFlex  source_string='LeftWristFlex'  names_length=16
      settings: SourceProductName=Sacros Robotics Toolbox
  Sarcos: Get Jacobian12 : RoboticsCode/Sarcos: Get Jacobian  urdfpath='XT_PRU_noHands.urdf'  source=LeftWrist6DOFLC_noHand  source_string='LeftWrist6DOFLC_noHand'  names_length=16
      settings: SourceProductName=Sacros Robotics Toolbox
  Sarcos: Get Jacobian13 : RoboticsCode/Sarcos: Get Jacobian  urdfpath='XT_PRU_noHands.urdf'  source=LeftLoadPointA  source_string='LeftLoadPointA'  names_length=16
      settings: SourceProductName=Sacros Robotics Toolbox
  Sarcos: Get Jacobian14 : RoboticsCode/Sarcos: Get Jacobian  urdfpath='XT_PRU_noHands.urdf'  source=LeftLoadPointB  source_string='LeftLoadPointB'  names_length=16
      settings: SourceProductName=Sacros Robotics Toolbox
  Sarcos: Get Jacobian15 : RoboticsCode/Sarcos: Get Jacobian  urdfpath='XT_PRU_noHands.urdf'  source=RightWristAbAd  source_string='RightWristAbAd'  names_length=16
      settings: SourceProductName=Sacros Robotics Toolbox
  Sarcos: Get Jacobian16 : RoboticsCode/Sarcos: Get Jacobian  urdfpath='XT_PRU_noHands.urdf'  source=RightWristFlex  source_string='RightWristFlex'  names_length=16
      settings: SourceProductName=Sacros Robotics Toolbox
  Sarcos: Get Jacobian17 : RoboticsCode/Sarcos: Get Jacobian  urdfpath='XT_PRU_noHands.urdf'  source=RightWrist6DOFLC_noHand  source_string='RightWrist6DOFLC_noHand'  names_length=16
      settings: SourceProductName=Sacros Robotics Toolbox
  Sarcos: Get Jacobian18 : RoboticsCode/Sarcos: Get Jacobian  urdfpath='XT_PRU_noHands.urdf'  source=RightLoadPointA  source_string='RightLoadPointA'  names_length=16
      settings: SourceProductName=Sacros Robotics Toolbox
  Sarcos: Get Jacobian19 : RoboticsCode/Sarcos: Get Jacobian  urdfpath='XT_PRU_noHands.urdf'  source=RightLoadPointB  source_string='RightLoadPointB'  names_length=16
      settings: SourceProductName=Sacros Robotics Toolbox
  Sarcos: Get Jacobian2 : RoboticsCode/Sarcos: Get Jacobian  urdfpath='XT_PRU_noHands.urdf'  source=TorsoForebend  source_string='TorsoForebend'  names_length=16
      settings: SourceProductName=Sacros Robotics Toolbox
  Sarcos: Get Jacobian20 : RoboticsCode/Sarcos: Get Jacobian  urdfpath='XT_PRU_noHands.urdf'  source=RightShoulderAbAd  source_string='RightShoulderAbAd'  names_length=16
      settings: SourceProductName=Sacros Robotics Toolbox
  Sarcos: Get Jacobian21 : RoboticsCode/Sarcos: Get Jacobian  urdfpath='XT_PRU_noHands.urdf'  source=RightShoulderFlex  source_string='RightShoulderFlex'  names_length=16
      settings: SourceProductName=Sacros Robotics Toolbox
  Sarcos: Get Jacobian22 : RoboticsCode/Sarcos: Get Jacobian  urdfpath='XT_PRU_noHands.urdf'  source=RightHumeralRotate  source_string='RightHumeralRotate'  names_length=16
      settings: SourceProductName=Sacros Robotics Toolbox
  Sarcos: Get Jacobian23 : RoboticsCode/Sarcos: Get Jacobian  urdfpath='XT_PRU_noHands.urdf'  source=RightElbowFlex  source_string='RightElbowFlex'  names_length=16
      settings: SourceProductName=Sacros Robotics Toolbox
  Sarcos: Get Jacobian24 : RoboticsCode/Sarcos: Get Jacobian  urdfpath='XT_PRU_noHands.urdf'  source=RightWristRotate  source_string='RightWristRotate'  names_length=16
      settings: SourceProductName=Sacros Robotics Toolbox
  Sarcos: Get Jacobian3 : RoboticsCode/Sarcos: Get Jacobian  urdfpath='XT_PRU_noHands.urdf'  source=CameraPan  source_string='CameraPan'  names_length=16
      settings: SourceProductName=Sacros Robotics Toolbox
  Sarcos: Get Jacobian4 : RoboticsCode/Sarcos: Get Jacobian  urdfpath='XT_PRU_noHands.urdf'  source=CameraTilt  source_string='CameraTilt'  names_length=16
      settings: SourceProductName=Sacros Robotics Toolbox
  Sarcos: Get Jacobian5 : RoboticsCode/Sarcos: Get Jacobian  urdfpath='XT_PRU_noHands.urdf'  source=LeftShoulderAbAd  source_string='LeftShoulderAbAd'  names_length=16
      settings: SourceProductName=Sacros Robotics Toolbox
  Sarcos: Get Jacobian6 : RoboticsCode/Sarcos: Get Jacobian  urdfpath='XT_PRU_noHands.urdf'  source=LeftShoulderFlex  source_string='LeftShoulderFlex'  names_length=16
      settings: SourceProductName=Sacros Robotics Toolbox
  Sarcos: Get Jacobian7 : RoboticsCode/Sarcos: Get Jacobian  urdfpath='XT_PRU_noHands.urdf'  source=LeftHumeralRotate  source_string='LeftHumeralRotate'  names_length=16
      settings: SourceProductName=Sacros Robotics Toolbox
  Sarcos: Get Jacobian8 : RoboticsCode/Sarcos: Get Jacobian  urdfpath='XT_PRU_noHands.urdf'  source=LeftElbowFlex  source_string='LeftElbowFlex'  names_length=16
      settings: SourceProductName=Sacros Robotics Toolbox
  Sarcos: Get Jacobian9 : RoboticsCode/Sarcos: Get Jacobian  urdfpath='XT_PRU_noHands.urdf'  source=LeftWristRotate  source_string='LeftWristRotate'  names_length=16
      settings: SourceProductName=Sacros Robotics Toolbox
  wires:
  q/1 -> Sarcos: Get Jacobian1/1, Sarcos: Get Jacobian2/1, Sarcos: Get Jacobian3/1, Sarcos: Get Jacobian4/1, Sarcos: Get Jacobian/1, Sarcos: Get Jacobian5/1, Sarcos: Get Jacobian14/1, Sarcos: Get Jacobian13/1, Sarcos: Get Jacobian12/1, Sarcos: Get Jacobian11/1, Sarcos: Get Jacobian10/1, Sarcos: Get Jacobian9/1, Sarcos: Get Jacobian8/1, Sarcos: Get Jacobian7/1, Sarcos: Get Jacobian6/1, Sarcos: Get Jacobian21/1, Sarcos: Get Jacobian22/1, Sarcos: Get Jacobian23/1, Sarcos: Get Jacobian24/1, Sarcos: Get Jacobian15/1, Sarcos: Get Jacobian16/1, Sarcos: Get Jacobian17/1, Sarcos: Get Jacobian18/1, Sarcos: Get Jacobian19/1, Sarcos: Get Jacobian20/1
  Sarcos: Get Jacobian/1 -> Display3/1  "Base"
  Sarcos: Get Jacobian1/1 -> Display1/1  "TorsoRotate"
  Sarcos: Get Jacobian2/1 -> Display4/1  "TorsoForebend"
  Sarcos: Get Jacobian3/1 -> Display2/1
  Sarcos: Get Jacobian4/1 -> Display5/1  "CameraTilt"
  Sarcos: Get Jacobian5/1 -> Display8/1  "LeftShoulderAbAd"
  Sarcos: Get Jacobian6/1 -> Display6/1  "LeftShoulderFlex"
  Sarcos: Get Jacobian7/1 -> Display9/1  "LeftHumeralRotate"
  Sarcos: Get Jacobian8/1 -> Display7/1  "LeftElbowFlex"
  Sarcos: Get Jacobian9/1 -> Display10/1  "LeftWristRotate"
  Sarcos: Get Jacobian10/1 -> Display14/1  "LeftWristAbAd"
  Sarcos: Get Jacobian11/1 -> Display12/1  "LeftWristFlex"
  Sarcos: Get Jacobian12/1 -> Display15/1  "LeftWrist6DOFLC_noHand"
  Sarcos: Get Jacobian13/1 -> Display13/1  "LeftLoadPointA"
  Sarcos: Get Jacobian14/1 -> Display11/1  "LeftLoadPointB"
  Sarcos: Get Jacobian20/1 -> Display24/1  "RightShoulderAbAd"
  Sarcos: Get Jacobian21/1 -> Display22/1  "RightShoulderFlex"
  Sarcos: Get Jacobian22/1 -> Display25/1
  Sarcos: Get Jacobian23/1 -> Display23/1  "RightElbowFlex"
  Sarcos: Get Jacobian24/1 -> Display16/1  "RightWristRotate"
  Sarcos: Get Jacobian15/1 -> Display20/1  "RightWristAbAd"
  Sarcos: Get Jacobian16/1 -> Display18/1  "RightWristFlex"
  Sarcos: Get Jacobian17/1 -> Display21/1  "RightWrist6DOFLC_noHand"
  Sarcos: Get Jacobian18/1 -> Display19/1  "RightLoadPointA"
  Sarcos: Get Jacobian19/1 -> Display17/1  "RightLoadPointB"
